simulink model "PMSMdetailTestbench"  (R2022b)
settings: Solver=ode1be  StartTime=0.0  StopTime=400  FixedStep=electricDrive.PmsmControlParams.Ts  RelTol=1e-3  EnableMultiTasking=on
PreLoadFcn:
  | PMSMSystemParamsPopl;
  | load WaterProperties.mat;
  | PMSMthermalParams;
StopFcn:
  | ee_addSimlogTimeStamp(bdroot)
undefined symbols (not defined in the file): electricDrive, p
libraries: fl_lib x71, nesl_utility x25, fl_ps_legacy_lib x23, ee_lib x4, eeTransforms x2, batteryecm_lib x1, autolibshared x1, eePmsmCurrentController x1, eePmsmFwController x1, simulink x1, eePmsmCurrentReferenceGen x1, eeVelocityController x1
(part 2 of 2)

== system PMSMdetailTestbench/Cooling System/Sensing Temperature ==
  Pressure & Temperature Sensor (TL) : fl_lib/Thermal Liquid/Sensors/Pressure & Temperature Sensor (TL)
      settings: InternalSimscapePortConfiguration="{\"Bottom\":[],\"Left\":[{\"id\":\"A\",\"label\":\"A\",\"type\":\"foundation.thermal_liquid.thermal_liquid\"}],\"Right\":[{\"id\":\"B\",\"label\":\"B\",\"type\":\"foundation.thermal_liquid.thermal_liquid\"},{\"id\":\"P\",\"label\":\"P\",\"type\":\"output\"},{\"id\":\"T\",\"label\":\"T\",\"type\":\"output\"}],\"Top\":[]}"
  TLRef : fl_lib/Thermal Liquid/Elements/Absolute Reference (TL)
  T : PMIOPort  Side=Right
  A : PMIOPort  Port=2  Side=Left
  connections:
  Pressure & Temperature Sensor (TL)/RConn3 -- T/RConn1
  TLRef/LConn1 -- Pressure & Temperature Sensor (TL)/RConn1
  A/RConn1 -- Pressure & Temperature Sensor (TL)/LConn1

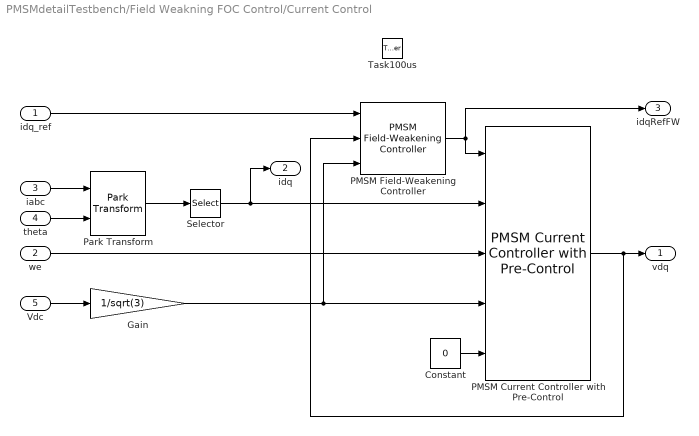
== system PMSMdetailTestbench/Field Weakning FOC Control/Current Control ==
  idq_ref : Inport
  we : Inport  Port=2
  iabc : Inport  Port=3
  theta : Inport  Port=4
  Vdc : Inport  Port=5
  Task100us : TriggerPort  TriggerType=function-call  VariantControl=Variant  PortDimensions=1
  Constant : Constant  Value=0  SampleTime=-1
  Gain : Gain  Gain=1/sqrt(3)
  PMSM Current Controller with Pre-Control : eePmsmCurrentController/PMSM Current Controller with Pre-Control  Kp_id=electricDrive.PmsmControlParams.Kp_id  Ki_id=electricDrive.PmsmControlParams.Ki_id  Kaw_id=1  Kp_iq=electricDrive.PmsmControlParams.Kp_iq  Ki_iq=electricDrive.PmsmControlParams.Ki_iq  Kaw_iq=1  Ts=-1  Tsd=electricDrive.PmsmControlParams.Tsi  AxisPrio=Q-axis  ActZC=on  ActFF=on  idVect=[-200, 0, 200]  iqVect=[-200, 0, 200]  LdMatrix=electricDrive.Ld * ones(3, 3)  LqMatrix=electricDrive.Lq * ones(3, 3)  psimMatrix=electricDrive.PmsmControlParams.psim * ones(3, 3)
  PMSM Field-Weakening Controller : eePmsmFwController/PMSM Field-Weakening Controller  Mth=0.95  Kfw=electricDrive.PmsmControlParams.Ki_fw  Kaw=electricDrive.PmsmControlParams.Kaw_fw  Ts=-1
  Park Transform : eeTransforms/Park Transform  AxisAlignment=Q-axis  PowerInvariant=off
  Selector : Selector  InputPortWidth=3  IndexOptions=Index vector (dialog)  Indices=[1 2]  OutputSizes=1
  vdq : Outport  VectorParamsAs1DForOutWhenUnconnected=off
  idq : Outport  Port=2  VectorParamsAs1DForOutWhenUnconnected=off
  idqRefFW : Outport  Port=3  VectorParamsAs1DForOutWhenUnconnected=off
  wires:
  Vdc/1 -> Gain/1
  iabc/1 -> Park Transform/1
  we/1 -> PMSM Current Controller with Pre-Control/3
  theta/1 -> Park Transform/2
  Constant/1 -> PMSM Current Controller with Pre-Control/5
  Selector/1 -> PMSM Current Controller with Pre-Control/2, idq/1
  Gain/1 -> PMSM Field-Weakening Controller/3, PMSM Current Controller with Pre-Control/4
  Park Transform/1 -> Selector/1
  PMSM Field-Weakening Controller/1 -> idqRefFW/1, PMSM Current Controller with Pre-Control/1
  PMSM Current Controller with Pre-Control/1 -> PMSM Field-Weakening Controller/2, vdq/1
  idq_ref/1 -> PMSM Field-Weakening Controller/1

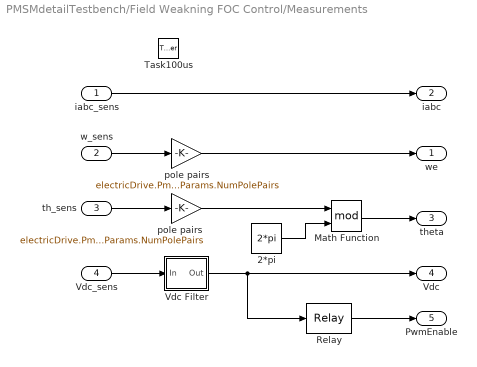
== system PMSMdetailTestbench/Field Weakning FOC Control/Measurements ==
  iabc_sens : Inport
  w_sens : Inport  Port=2
  th_sens : Inport  Port=3
  Vdc_sens : Inport  Port=4
  Task100us : TriggerPort  TriggerType=function-call  VariantControl=Variant  PortDimensions=1
  2*pi : Constant  Value=2*pi  SampleTime=-1
  Math Function : Math  Operator=mod  SignedPower=on
  Relay : Relay  OnSwitchValue=200  OffSwitchValue=100
  Vdc Filter : Subsystem  mask(Discrete first-order filter (Low-pass)){T=0.005, Ts=1e-4}
      mask prompts: T "Time constant (s):"; Ts "Sample time (s):"
      mask help: This block implements a discrete low-pass filter. To calculate the coefficients, the block discretises a continuous low-pass filter using the Tustin method.
      mask init:
      | num = [ Ts/(2*T + Ts), Ts/(2*T + Ts)];
      | den = [ 1, -(2*T - Ts)/(2*T + Ts)];
  pole pairs : Gain  Gain=electricDrive.PmsmParams.NumPolePairs
  "pole pairs " : Gain  Gain=electricDrive.PmsmParams.NumPolePairs
  we : Outport  VectorParamsAs1DForOutWhenUnconnected=off
  iabc : Outport  Port=2  VectorParamsAs1DForOutWhenUnconnected=off
  theta : Outport  Port=3  VectorParamsAs1DForOutWhenUnconnected=off
  Vdc : Outport  Port=4  VectorParamsAs1DForOutWhenUnconnected=off
  PwmEnable : Outport  Port=5  VectorParamsAs1DForOutWhenUnconnected=off
  wires:
  pole pairs/1 -> we/1
  Vdc_sens/1 -> Vdc Filter/1(In)
  th_sens/1 -> "pole pairs "/1
  w_sens/1 -> pole pairs/1
  iabc_sens/1 -> iabc/1
  "pole pairs "/1 -> Math Function/1
  2*pi/1 -> Math Function/2
  Math Function/1 -> theta/1
  Relay/1 -> PwmEnable/1
  Vdc Filter/1(Out) -> Relay/1, Vdc/1

== system PMSMdetailTestbench/Field Weakning FOC Control/Outer Loop Control ==
  RPMReq : Inport
  we : Inport  Port=2
  Vdc : Inport  Port=3
  Task1ms : TriggerPort  TriggerType=function-call  VariantControl=Variant  PortDimensions=1
  Constant : Constant  Value=0  SampleTime=-1
  PMSM Current Reference Generator : eePmsmCurrentReferenceGen/PMSM Current Reference Generator  Vnom=electricDrive.Vnom  Pmax=electricDrive.Pmax  Tmax=electricDrive.Tmax  Ts=-1  RefType=Zero d-axis control  rpmVec=[0, 3000]  TqVec=[-100, 0, 100]  VdcVec=[300, 350]  PWMMode=SVM: space vector modulation  ModFactor=1  idMatrix=zeros(2,3,2)  iqMatrix=zeros(2,3,2)  p=electricDrive.PmsmParams.NumPolePairs  psim=electricDrive.PmsmControlParams.psim  Ld=0.00024  Lq=0.00029  Rs=0.01  RefExpEnable=0
  Velocity Controller : eeVelocityController/Velocity Controller  CtrlType=P-PI control  Kp_w=electricDrive.PmsmControlParams.Kp_omega  Ki_w=electricDrive.PmsmControlParams.Ki_omega  Kv_w=electricDrive.PmsmControlParams.Kp_omega  Kaw_w=100  Ts=-1  Tsd=electricDrive.PmsmControlParams.Tso  ActZC=on
  elec->mech : Gain  Gain=1/electricDrive.PmsmParams.NumPolePairs
  rpm->rad/s : Gain  Gain=(pi/30)
  idqRef : Outport  VectorParamsAs1DForOutWhenUnconnected=off
  Tq_ref : Outport  Port=2  VectorParamsAs1DForOutWhenUnconnected=off
  Tq_lim : Outport  Port=3  VectorParamsAs1DForOutWhenUnconnected=off
  wires:
  rpm->rad/s/1 -> Velocity Controller/1
  Velocity Controller/1 -> PMSM Current Reference Generator/1
  RPMReq/1 -> rpm->rad/s/1
  we/1 -> elec->mech/1
  Vdc/1 -> PMSM Current Reference Generator/3
  PMSM Current Reference Generator/2 -> Tq_ref/1, Velocity Controller/3
  PMSM Current Reference Generator/3 -> Tq_lim/1
  elec->mech/1 -> PMSM Current Reference Generator/2, Velocity Controller/2
  Constant/1 -> Velocity Controller/4
  PMSM Current Reference Generator/1 -> idqRef/1

== system PMSMdetailTestbench/Scopes/Modulation index ==
  vdq : Inport
  Vdc : Inport  Port=2
  Gain1 : Gain  Gain=1/sqrt(3)
  Math Function : Math  Operator=square  SignedPower=on
  Prevent division by 0 : Subsystem
  Product : Product  Inputs=*/
  Rate Transition4 : RateTransition  OutPortSampleTime=electricDrive.PmsmControlParams.Tsi
  Rate Transition5 : RateTransition  OutPortSampleTime=electricDrive.PmsmControlParams.Tsi
  Sqrt : Sqrt
  Sum of Elements : Sum  Inputs=+
  M : Outport  VectorParamsAs1DForOutWhenUnconnected=off
  wires:
  Sum of Elements/1 -> Sqrt/1
  Vdc/1 -> Rate Transition4/1
  Sqrt/1 -> Product/1
  Math Function/1 -> Sum of Elements/1
  Product/1 -> M/1
  Prevent division by 0/1(OUT) -> Product/2
  vdq/1 -> Rate Transition5/1
  Rate Transition4/1 -> Gain1/1
  Gain1/1 -> Prevent division by 0/1(IN)
  Rate Transition5/1 -> Math Function/1

== system PMSMdetailTestbench/Test Environment/Bus ==
  In : Inport
  Wi : Inport  Port=2
  Br : Inport  Port=3
  Bus Creator : BusCreator  Inputs=3
  b : Outport  VectorParamsAs1DForOutWhenUnconnected=off
  wires:
  Wi/1 -> Bus Creator/2  "Wind speed"
  Bus Creator/1 -> b/1
  Br/1 -> Bus Creator/3  "Brake pedal"
  In/1 -> Bus Creator/1  "Incline"

== system PMSMdetailTestbench/Vehicle Dynamics/Brake Torque ==
  Pedal : Inport
  Force for max pedal deflection : Gain  Gain=100
  Ideal Torque Sensor : fl_lib/Mechanical/Mechanical Sensors/Ideal Torque Sensor
  Ideal Torque Source : fl_lib/Mechanical/Mechanical Sources/Ideal Torque Source
  MRRef : fl_lib/Mechanical/Rotational Elements/Mechanical Rotational Reference
  PS-Simulink Converter : nesl_utility/PS-Simulink Converter  PhysicalDomain=network_engine_domain  SubClassName=ps_output  LeftPortType=input  RightPortType=output  PseudoPeriodic=off  Frequencies=[]  VectorFormat=inherit  Unit=inherit  AffineConversion=off
  Paddle travel : TransferFcn  Numerator=[4]  Denominator=[2 1]
  Scope : Scope
  Simulink-PS Converter1 : nesl_utility/Simulink-PS Converter  PhysicalDomain=network_engine_domain  SubClassName=ps_input  LeftPortType=input  RightPortType=output  PseudoPeriodic=off  Frequencies=[]  NoiseDistribution=none  NoiseParameters=[]  Unit=N*m  AffineConversion=off  FilteringAndDerivatives=zero  SimscapeFilterOrder=1  InputFilterTimeConstant=0.001  UdotUserProvided=1
  Torque per unit brake pedal force : Gain  Gain=7.5
  R : PMIOPort  Side=Right
  wires:
  Pedal/1 -> Paddle travel/1
  Force for max pedal deflection/1 -> Torque per unit brake pedal force/1
  PS-Simulink Converter/1 -> Scope/1
  Torque per unit brake pedal force/1 -> Simulink-PS Converter1/1
  Paddle travel/1 -> Force for max pedal deflection/1
  connections:
  MRRef/LConn1 -- Ideal Torque Source/RConn2
  Ideal Torque Source/LConn1 -- Ideal Torque Sensor/RConn1
  Ideal Torque Source/RConn1 -- Simulink-PS Converter1/RConn1
  Ideal Torque Sensor/LConn1 -- R/RConn1
  PS-Simulink Converter/LConn1 -- Ideal Torque Sensor/RConn2

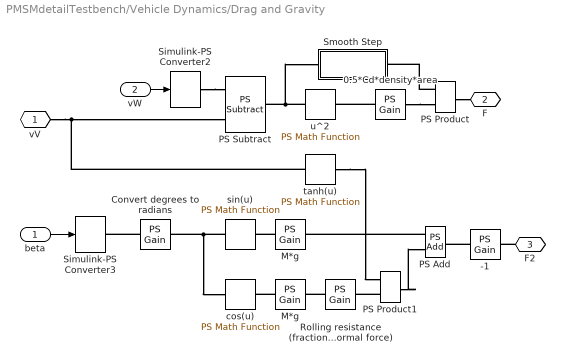
== system PMSMdetailTestbench/Vehicle Dynamics/Drag and Gravity ==
  beta : Inport
  vW : Inport  Port=2
  " M*g " : fl_ps_legacy_lib/Legacy Physical Signals/Functions/PS Gain  gain=electricDrive.VehicleParams.vehicle_mass*electricDrive.gravity
  -1 : fl_ps_legacy_lib/Legacy Physical Signals/Functions/PS Gain  gain=-1
  0.5*Cd*density*area : fl_ps_legacy_lib/Legacy Physical Signals/Functions/PS Gain  gain=0.5*electricDrive.drag_coefficient*electricDrive.air_density*electricDrive.VehicleParams.Frontalarea
  "Convert degrees to radians " : fl_ps_legacy_lib/Legacy Physical Signals/Functions/PS Gain  gain=pi/180
  M*g : fl_ps_legacy_lib/Legacy Physical Signals/Functions/PS Gain  gain=electricDrive.VehicleParams.vehicle_mass*electricDrive.gravity
  PS Add : fl_ps_legacy_lib/Legacy Physical Signals/Functions/PS Add
      settings: InternalSimscapePortConfiguration="{\"Bottom\":[],\"Left\":[{\"id\":\"I1\",\"label\":\"\",\"type\":\"input\"},{\"id\":\"I2\",\"label\":\"\",\"type\":\"input\"}],\"Right\":[{\"id\":\"O\",\"label\":\"\",\"type\":\"output\"}],\"Top\":[]}"
  PS Product : fl_ps_legacy_lib/Legacy Physical Signals/Functions/PS Product
  PS Product1 : fl_ps_legacy_lib/Legacy Physical Signals/Functions/PS Product
  PS Subtract : fl_ps_legacy_lib/Legacy Physical Signals/Functions/PS Subtract
  "Rolling resistance (fraction of normal force) " : fl_ps_legacy_lib/Legacy Physical Signals/Functions/PS Gain  gain=electricDrive.VehicleParams.rolling_res_ratio
  Simulink-PS Converter2 : nesl_utility/Simulink-PS Converter  PhysicalDomain=network_engine_domain  SubClassName=ps_input  LeftPortType=input  RightPortType=output  PseudoPeriodic=off  Frequencies=[]  NoiseDistribution=none  NoiseParameters=[]  Unit=N*m  AffineConversion=off  FilteringAndDerivatives=zero  SimscapeFilterOrder=1  InputFilterTimeConstant=0.001  UdotUserProvided=1
  Simulink-PS Converter3 : nesl_utility/Simulink-PS Converter  PhysicalDomain=network_engine_domain  SubClassName=ps_input  LeftPortType=input  RightPortType=output  PseudoPeriodic=off  Frequencies=[]  NoiseDistribution=none  NoiseParameters=[]  Unit=N*m  AffineConversion=off  FilteringAndDerivatives=zero  SimscapeFilterOrder=1  InputFilterTimeConstant=0.001  UdotUserProvided=1
  Smooth Step : Subsystem
  cos(u) : fl_ps_legacy_lib/Legacy Physical Signals/Functions/PS Math Function  fcn_choice=2
      settings: InternalSimscapePortConfiguration="{\"Bottom\":[],\"Left\":[{\"id\":\"I\",\"label\":\"\",\"type\":\"input\"}],\"Right\":[{\"id\":\"O\",\"label\":\"\",\"type\":\"output\"}],\"Top\":[]}"
  sin(u) : fl_ps_legacy_lib/Legacy Physical Signals/Functions/PS Math Function  fcn_choice=1
      settings: InternalSimscapePortConfiguration="{\"Bottom\":[],\"Left\":[{\"id\":\"I\",\"label\":\"\",\"type\":\"input\"}],\"Right\":[{\"id\":\"O\",\"label\":\"\",\"type\":\"output\"}],\"Top\":[]}"
  tanh(u) : fl_ps_legacy_lib/Legacy Physical Signals/Functions/PS Math Function  fcn_choice=10
      settings: InternalSimscapePortConfiguration="{\"Bottom\":[],\"Left\":[{\"id\":\"I\",\"label\":\"\",\"type\":\"input\"}],\"Right\":[{\"id\":\"O\",\"label\":\"\",\"type\":\"output\"}],\"Top\":[]}"
  u^2 : fl_ps_legacy_lib/Legacy Physical Signals/Functions/PS Math Function  fcn_choice=7
      settings: InternalSimscapePortConfiguration="{\"Bottom\":[],\"Left\":[{\"id\":\"I\",\"label\":\"\",\"type\":\"input\"}],\"Right\":[{\"id\":\"O\",\"label\":\"\",\"type\":\"output\"}],\"Top\":[]}"
  vV : PMIOPort  Side=Left
  F : PMIOPort  Port=2  Side=Left
  F2 : PMIOPort  Port=3  Side=Left
  wires:
  vW/1 -> Simulink-PS Converter2/1
  beta/1 -> Simulink-PS Converter3/1
  connections:
  vV/RConn1 -- tanh(u)/LConn1 -- PS Subtract/LConn1
  Simulink-PS Converter2/RConn1 -- PS Subtract/LConn2
  u^2/LConn1 -- Smooth Step/LConn1 -- PS Subtract/RConn1
  0.5*Cd*density*area/LConn1 -- u^2/RConn1
  0.5*Cd*density*area/RConn1 -- PS Product/LConn2
  PS Product/RConn1 -- F/RConn1
  PS Product/LConn1 -- Smooth Step/RConn1
  "Convert degrees to radians "/LConn1 -- Simulink-PS Converter3/RConn1
  sin(u)/LConn1 -- "Convert degrees to radians "/RConn1 -- cos(u)/LConn1
  M*g/LConn1 -- sin(u)/RConn1
  " M*g "/LConn1 -- cos(u)/RConn1
  "Rolling resistance (fraction of normal force) "/LConn1 -- " M*g "/RConn1
  PS Product1/LConn2 -- "Rolling resistance (fraction of normal force) "/RConn1
  PS Add/LConn1 -- M*g/RConn1
  PS Product1/RConn1 -- PS Add/LConn2
  -1/LConn1 -- PS Add/RConn1
  F2/RConn1 -- -1/RConn1
  tanh(u)/RConn1 -- PS Product1/LConn1

== system PMSMdetailTestbench/Vehicle Dynamics/Sensing Speed ==
  MTRef : fl_lib/Mechanical/Translational Elements/Mechanical Translational Reference
  Motion Sensor : fl_lib/Mechanical/Mechanical Sensors/Ideal Translational Motion Sensor  reference=foundation.enum.MeasurementReference.difference  acceleration_port=false  velocity_port=true  position_port=true  offset=0 m
  PS-Simulink Converter3 : nesl_utility/PS-Simulink Converter  PhysicalDomain=network_engine_domain  SubClassName=ps_output  LeftPortType=input  RightPortType=output  PseudoPeriodic=off  Frequencies=[]  VectorFormat=1-D array  Unit=mph  AffineConversion=off
  R : PMIOPort  Side=Left
  w : PMIOPort  Port=2  Side=Right
  tag scope: vSpd=global
  wires:
  PS-Simulink Converter3/1 -> [vSpd]  "Vehicle Speed"
  connections:
  R/RConn1 -- Motion Sensor/LConn1
  MTRef/LConn1 -- Motion Sensor/RConn1
  Motion Sensor/RConn2 -- PS-Simulink Converter3/LConn1 -- w/RConn1

== system PMSMdetailTestbench/ Motor Thermal/Air_HTC_calculation/Rotor side  HTC ==
  Abs : Abs  SaturateOnIntegerOverflow=off
  Gain4 : Gain  Gain=0.75
  PS-Simulink Converter5 : nesl_utility/PS-Simulink Converter  PhysicalDomain=network_engine_domain  SubClassName=ps_output  LeftPortType=input  RightPortType=output  PseudoPeriodic=off  Frequencies=[]  VectorFormat=inherit  Unit=inherit  AffineConversion=off
  Sqrt : Sqrt
  Unit Delay3 : UnitDelay  SampleTime=-1  HasFrameUpgradeWarning=on
  RPM : PMIOPort  Side=Left
  Output : Outport
  wires:
  Gain4/1 -> Output/1
  Sqrt/1 -> Gain4/1
  Unit Delay3/1 -> Abs/1
  Abs/1 -> Sqrt/1
  PS-Simulink Converter5/1 -> Unit Delay3/1
  connections:
  RPM/RConn1 -- PS-Simulink Converter5/LConn1

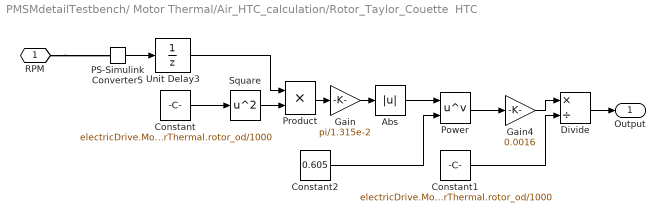
== system PMSMdetailTestbench/ Motor Thermal/Air_HTC_calculation/Rotor_Taylor_Couette  HTC ==
  Abs : Abs  SaturateOnIntegerOverflow=off
  Constant : Constant  Value=electricDrive.MotorThermal.rotor_od/1000
  Constant1 : Constant  Value=electricDrive.MotorThermal.rotor_od/1000
  Constant2 : Constant  Value=0.605
  Divide : Product  Inputs=*/
  Gain : Gain  Gain=pi/1.315e-2
  Gain4 : Gain  Gain=0.0016
  PS-Simulink Converter5 : nesl_utility/PS-Simulink Converter  PhysicalDomain=network_engine_domain  SubClassName=ps_output  LeftPortType=input  RightPortType=output  PseudoPeriodic=off  Frequencies=[]  VectorFormat=inherit  Unit=inherit  AffineConversion=off
  Power : Math  Operator=pow
  Product : Product
  Square : Math  Operator=square
  Unit Delay3 : UnitDelay  SampleTime=-1  HasFrameUpgradeWarning=on
  RPM : PMIOPort  Side=Left
  Output : Outport
  wires:
  Power/1 -> Gain4/1
  Unit Delay3/1 -> Product/1
  PS-Simulink Converter5/1 -> Unit Delay3/1
  Product/1 -> Gain/1
  Square/1 -> Product/2
  Constant/1 -> Square/1
  Gain4/1 -> Divide/1
  Constant1/1 -> Divide/2
  Divide/1 -> Output/1
  Gain/1 -> Abs/1
  Abs/1 -> Power/1
  Constant2/1 -> Power/2
  connections:
  RPM/RConn1 -- PS-Simulink Converter5/LConn1

== system PMSMdetailTestbench/ Motor Thermal/Loss Re-distribution/Iron Loss ==
  Hmot_s : Inport
  Gain1 : Gain  Gain=electricDrive.MotorThermal.vFractBridge
  Gain2 : Gain  Gain=electricDrive.MotorThermal.vFractTooth
  Unit Delay : UnitDelay  SampleTime=-1  HasFrameUpgradeWarning=on
  st : Outport
  rt : Outport  Port=2
  wires:
  Hmot_s/1 -> Gain1/1, Unit Delay/1  "Iron_Loss"
  Gain1/1 -> rt/1
  Unit Delay/1 -> Gain2/1
  Gain2/1 -> st/1

== system PMSMdetailTestbench/ Motor Thermal/Loss Re-distribution/Subsystem ==
  Heat Flow Rate Sensor : fl_lib/Thermal/Thermal Sensors/Heat Flow Rate Sensor
  PS-Simulink Converter1 : nesl_utility/PS-Simulink Converter  PhysicalDomain=network_engine_domain  SubClassName=ps_output  LeftPortType=input  RightPortType=output  PseudoPeriodic=off  Frequencies=[]  VectorFormat=inherit  Unit=inherit  AffineConversion=off
  Temperature Source : fl_lib/Thermal/Thermal Sources/Temperature Source  temperature=298.15 K
  Hmot : PMIOPort  Side=Left
  Hmot_Cu : Outport
  wires:
  PS-Simulink Converter1/1 -> Hmot_Cu/1
  connections:
  Heat Flow Rate Sensor/RConn1 -- PS-Simulink Converter1/LConn1
  Hmot/RConn1 -- Heat Flow Rate Sensor/LConn1
  Temperature Source/LConn1 -- Heat Flow Rate Sensor/RConn2

== system PMSMdetailTestbench/ Motor Thermal/Loss Re-distribution/Subsystem1 ==
  Heat Flow Rate Sensor : fl_lib/Thermal/Thermal Sensors/Heat Flow Rate Sensor
  PS-Simulink Converter1 : nesl_utility/PS-Simulink Converter  PhysicalDomain=network_engine_domain  SubClassName=ps_output  LeftPortType=input  RightPortType=output  PseudoPeriodic=off  Frequencies=[]  VectorFormat=inherit  Unit=inherit  AffineConversion=off
  Temperature Source : fl_lib/Thermal/Thermal Sources/Temperature Source  temperature=298.15 K
  Hmot : PMIOPort  Side=Left
  Hmot_Fe : Outport
  wires:
  PS-Simulink Converter1/1 -> Hmot_Fe/1
  connections:
  Heat Flow Rate Sensor/RConn1 -- PS-Simulink Converter1/LConn1
  Hmot/RConn1 -- Heat Flow Rate Sensor/LConn1
  Temperature Source/LConn1 -- Heat Flow Rate Sensor/RConn2

== system PMSMdetailTestbench/ Motor Thermal/Loss Re-distribution/Subsystem2 ==
  Heat Flow Rate Sensor : fl_lib/Thermal/Thermal Sensors/Heat Flow Rate Sensor
  PS-Simulink Converter1 : nesl_utility/PS-Simulink Converter  PhysicalDomain=network_engine_domain  SubClassName=ps_output  LeftPortType=input  RightPortType=output  PseudoPeriodic=off  Frequencies=[]  VectorFormat=inherit  Unit=inherit  AffineConversion=off
  Temperature Source : fl_lib/Thermal/Thermal Sources/Temperature Source  temperature=298.15 K
  Hmot : PMIOPort  Side=Left
  Hmot_Cu : Outport
  wires:
  PS-Simulink Converter1/1 -> Hmot_Cu/1
  connections:
  Heat Flow Rate Sensor/RConn1 -- PS-Simulink Converter1/LConn1
  Hmot/RConn1 -- Heat Flow Rate Sensor/LConn1
  Temperature Source/LConn1 -- Heat Flow Rate Sensor/RConn2

== system PMSMdetailTestbench/ Motor Thermal/Loss Re-distribution/Subsystem3 ==
  Heat Flow Rate Sensor : fl_lib/Thermal/Thermal Sensors/Heat Flow Rate Sensor
  PS-Simulink Converter1 : nesl_utility/PS-Simulink Converter  PhysicalDomain=network_engine_domain  SubClassName=ps_output  LeftPortType=input  RightPortType=output  PseudoPeriodic=off  Frequencies=[]  VectorFormat=inherit  Unit=inherit  AffineConversion=off
  Temperature Source : fl_lib/Thermal/Thermal Sources/Temperature Source  temperature=298.15 K
  Hmot : PMIOPort  Side=Left
  Hmot_Cu : Outport
  wires:
  PS-Simulink Converter1/1 -> Hmot_Cu/1
  connections:
  Heat Flow Rate Sensor/RConn1 -- PS-Simulink Converter1/LConn1
  Hmot/RConn1 -- Heat Flow Rate Sensor/LConn1
  Temperature Source/LConn1 -- Heat Flow Rate Sensor/RConn2

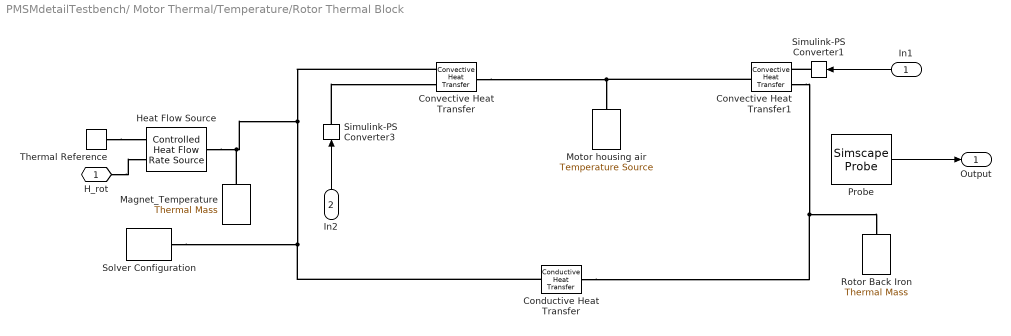
== system PMSMdetailTestbench/ Motor Thermal/Temperature/Rotor Thermal Block ==
  In1 : Inport
  In2 : Inport  Port=2
  Conductive Heat Transfer : fl_lib/Thermal/Thermal Elements/Conductive Heat Transfer  thermal_type=foundation.enum.ConstantVariableTabulated.Constant  wall_geometry=foundation.enum.ConductionWallGeometry.Cylindrical  area=1e-4 m^2  thickness=0.1 m  d_in=0.005 m  d_out=electricDrive.MotorThermal.rotor_od m  L=electricDrive.MotorThermal.rotorStackLength m  th_cond_min=10 W/(K*m)  th_cond=electricDrive.IronThConductivity W/(K*m)  th_cond_TLU=[413, 401, 392, 383, 371, 357, 342] W/(K*m)  temp_TLU=[200, 273, 400, 600, 800, 1000, 1200] K  T_specify=off  T_priority=None  T=0 K  T_nominal_specify=off  T_nominal_unit=K  T_nominal_value=1  Q_specify=off  Q_priority=None  Q=0 W  Q_nominal_specify=off  Q_nominal_unit=W  Q_nominal_value=1
  Convective Heat Transfer : fl_lib/Thermal/Thermal Elements/Convective Heat Transfer  thermal_type=foundation.enum.constant_variable.variable  area=electricDrive.MotorThermal.RotorAreaCyl m^2  heat_tr_coeff=10 W/(K*m^2)  min_heat_tr_coeff=1e-3 W/(K*m^2)  T_specify=off  T_priority=None  T=0 K  T_nominal_specify=off  T_nominal_unit=K  T_nominal_value=1  Q_specify=off  Q_priority=None  Q=0 W  Q_nominal_specify=off  Q_nominal_unit=W  Q_nominal_value=1
      settings: InternalSimscapePortConfiguration="{\"Bottom\":[],\"Left\":[{\"id\":\"A\",\"label\":\"A\",\"type\":\"foundation.thermal.thermal\"},{\"id\":\"var_heat_tr_coeff\",\"label\":\"K\",\"type\":\"input\"}],\"Right\":[{\"id\":\"B\",\"label\":\"B\",\"type\":\"foundation.thermal.thermal\"}],\"Top\":[]}"
  Convective Heat Transfer1 : fl_lib/Thermal/Thermal Elements/Convective Heat Transfer  thermal_type=foundation.enum.constant_variable.variable  area=electricDrive.MotorThermal.RotorAreaER m^2  heat_tr_coeff=20 W/(K*m^2)  min_heat_tr_coeff=1e-3 W/(K*m^2)  T_specify=off  T_priority=None  T=0 K  T_nominal_specify=off  T_nominal_unit=K  T_nominal_value=1  Q_specify=off  Q_priority=None  Q=0 W  Q_nominal_specify=off  Q_nominal_unit=W  Q_nominal_value=1
      settings: InternalSimscapePortConfiguration="{\"Bottom\":[],\"Left\":[{\"id\":\"A\",\"label\":\"A\",\"type\":\"foundation.thermal.thermal\"},{\"id\":\"var_heat_tr_coeff\",\"label\":\"K\",\"type\":\"input\"}],\"Right\":[{\"id\":\"B\",\"label\":\"B\",\"type\":\"foundation.thermal.thermal\"}],\"Top\":[]}"
  Heat Flow Source : fl_lib/Thermal/Thermal Sources/Controlled Heat Flow Rate Source
  "Magnet_Temperature " : fl_lib/Thermal/Thermal Elements/Thermal Mass  mass=electricDrive.MotorThermal.Bridgemass kg  sp_heat=447 J/(K*kg)  num_ports=foundation.enum.numPorts2.one  T_specify=on  T_priority=High  T=298.15 K  T_nominal_specify=off  T_nominal_unit=K  T_nominal_value=1  Q_specify=off  Q_priority=None  Q=0 W  Q_nominal_specify=off  Q_nominal_unit=W  Q_nominal_value=1
  Motor housing air : fl_lib/Thermal/Thermal Sources/Temperature Source  temperature=298.15 K
  Probe : SimscapeProbe  BoundBlock=1368  Variables={T}
  Rotor Back Iron : fl_lib/Thermal/Thermal Elements/Thermal Mass  mass=electricDrive.MotorThermal.RotorBackIronMass kg  sp_heat=447 J/(K*kg)  num_ports=foundation.enum.numPorts2.one  T_specify=on  T_priority=High  T=298.15 K  T_nominal_specify=off  T_nominal_unit=K  T_nominal_value=1  Q_specify=off  Q_priority=None  Q=0 W  Q_nominal_specify=off  Q_nominal_unit=W  Q_nominal_value=1
  Simulink-PS Converter1 : nesl_utility/Simulink-PS Converter  PhysicalDomain=network_engine_domain  SubClassName=ps_input  LeftPortType=input  RightPortType=output  PseudoPeriodic=off  Frequencies=[]  NoiseDistribution=none  NoiseParameters=[]  Unit=W/(K* m^2)  AffineConversion=off  FilteringAndDerivatives=provide  SimscapeFilterOrder=1  InputFilterTimeConstant=0.001  UdotUserProvided=0
  Simulink-PS Converter3 : nesl_utility/Simulink-PS Converter  PhysicalDomain=network_engine_domain  SubClassName=ps_input  LeftPortType=input  RightPortType=output  PseudoPeriodic=off  Frequencies=[]  NoiseDistribution=none  NoiseParameters=[]  Unit=W/(K* m^2)  AffineConversion=off  FilteringAndDerivatives=provide  SimscapeFilterOrder=1  InputFilterTimeConstant=0.001  UdotUserProvided=0
  Solver Configuration : nesl_utility/Solver Configuration  PhysicalDomain=network_engine_domain  SubClassName=solver  LeftPortType=input  RightPortType=generic  Tones=[]  Harmonics=[]  SimulateNoise=off  Profile=off  UseLocalSampling=off  EnableSwitchedLinearOptims=on  FrequencyDomain=off  UseCCode=off  RelTol=0.001  AbsTol=0.001  MinStep=1e-09  ToWorkspace=off  RevertToSquareIcSolve=off  NumHomotopyIterations=100  PhasorMode=off  PhasorModeNumHarmonics=1  ConsistencySolver=NEWTON_XTOL_AFTER_FTOL  IndexReductionMethod=DerivativeReplacement  DoDC=off  ResidualTolerance=1e-09  ConsistencyTolSource=GLOBAL  ConsistencyAbsTol=0.001  ConsistencyRelTol=0.001  ConsistencyTolFactor=0.001  UseLocalSolver=on  LocalSolverChoice=NE_BACKWARD_EULER_ADVANCER  ResolveIndetEquations=on  FunctionEvalNumThread=1  LocalSolverSampleTime=electricDrive.dt  DoFixedCost=on  MaxNonlinIter=3  MaxModeIter=2  ComputeImpulses=off  ImpulseIterations=2  LinearAlgebra=auto  LinearAlgebraNumThread=0  EquationFormulation=NE_TIME_EF  DelaysMemoryBudget=1024  AutomaticFiltering=on  FilteringTimeConstant=0.001  PartitionStorageMethod=AS_NEEDED  PartitionMemoryBudget=1024  PartitionMethod=ROBUST
  Thermal Reference : fl_lib/Thermal/Thermal Elements/Thermal Reference
  H_rot : PMIOPort  Side=Right
  Output : Outport
  wires:
  In2/1 -> Simulink-PS Converter3/1
  Probe/1 -> Output/1
  In1/1 -> Simulink-PS Converter1/1
  connections:
  Thermal Reference/LConn1 -- Heat Flow Source/RConn2
  Conductive Heat Transfer/RConn1 -- Convective Heat Transfer1/LConn1 -- Rotor Back Iron/LConn1
  Convective Heat Transfer1/RConn1 -- Convective Heat Transfer/RConn1 -- Motor housing air/LConn1
  Heat Flow Source/LConn1 -- Convective Heat Transfer/LConn1 -- Conductive Heat Transfer/LConn1 -- Solver Configuration/RConn1 -- "Magnet_Temperature "/LConn1
  Simulink-PS Converter3/RConn1 -- Convective Heat Transfer/LConn2
  H_rot/RConn1 -- Heat Flow Source/RConn1
  Simulink-PS Converter1/RConn1 -- Convective Heat Transfer1/LConn2

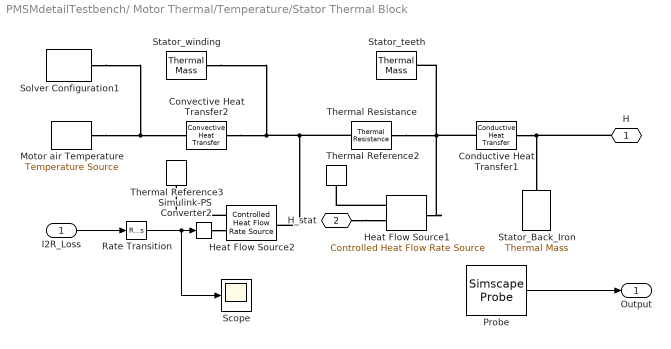
== system PMSMdetailTestbench/ Motor Thermal/Temperature/Stator Thermal Block ==
  I2R_Loss : Inport
  Conductive Heat Transfer1 : fl_lib/Thermal/Thermal Elements/Conductive Heat Transfer  thermal_type=foundation.enum.ConstantVariableTabulated.Constant  wall_geometry=foundation.enum.ConductionWallGeometry.Cylindrical  area=1e-4 m^2  thickness=0.1 m  d_in=electricDrive.MotorThermal.StatorRootDia m  d_out=electricDrive.MotorThermal.stator_od m  L=electricDrive.MotorThermal.rotorStackLength m  th_cond_min=10 W/(K*m)  th_cond=50 W/(K*m)  th_cond_TLU=[413, 401, 392, 383, 371, 357, 342] W/(K*m)  temp_TLU=[200, 273, 400, 600, 800, 1000, 1200] K  T_specify=off  T_priority=None  T=0 K  T_nominal_specify=off  T_nominal_unit=K  T_nominal_value=1  Q_specify=off  Q_priority=None  Q=0 W  Q_nominal_specify=off  Q_nominal_unit=W  Q_nominal_value=1
  Convective Heat Transfer2 : fl_lib/Thermal/Thermal Elements/Convective Heat Transfer  thermal_type=foundation.enum.constant_variable.constant  area=electricDrive.MotorThermal.StatorWindingOhArea m^2  heat_tr_coeff=1 W/(K*m^2)  min_heat_tr_coeff=1e-3 W/(K*m^2)  T_specify=off  T_priority=None  T=0 K  T_nominal_specify=off  T_nominal_unit=K  T_nominal_value=1  Q_specify=off  Q_priority=None  Q=0 W  Q_nominal_specify=off  Q_nominal_unit=W  Q_nominal_value=1
  Heat Flow Source1 : fl_lib/Thermal/Thermal Sources/Controlled Heat Flow Rate Source
  Heat Flow Source2 : fl_lib/Thermal/Thermal Sources/Controlled Heat Flow Rate Source
  Motor air Temperature : fl_lib/Thermal/Thermal Sources/Temperature Source  temperature=90 degC
  Probe : SimscapeProbe  BoundBlock=1401  Variables={T}
  Rate Transition : RateTransition
  Scope : Scope
  Simulink-PS Converter2 : nesl_utility/Simulink-PS Converter  PhysicalDomain=network_engine_domain  SubClassName=ps_input  LeftPortType=input  RightPortType=output  PseudoPeriodic=off  Frequencies=[]  NoiseDistribution=none  NoiseParameters=[]  Unit=W  AffineConversion=off  FilteringAndDerivatives=provide  SimscapeFilterOrder=1  InputFilterTimeConstant=0.001  UdotUserProvided=0
  Solver Configuration1 : nesl_utility/Solver Configuration  PhysicalDomain=network_engine_domain  SubClassName=solver  LeftPortType=input  RightPortType=generic  Tones=[]  Harmonics=[]  SimulateNoise=off  Profile=off  UseLocalSampling=off  EnableSwitchedLinearOptims=on  FrequencyDomain=off  UseCCode=off  RelTol=0.001  AbsTol=0.001  MinStep=1e-09  ToWorkspace=off  RevertToSquareIcSolve=off  NumHomotopyIterations=100  PhasorMode=off  PhasorModeNumHarmonics=1  ConsistencySolver=NEWTON_XTOL_AFTER_FTOL  IndexReductionMethod=DerivativeReplacement  DoDC=off  ResidualTolerance=1e-09  ConsistencyTolSource=GLOBAL  ConsistencyAbsTol=0.001  ConsistencyRelTol=0.001  ConsistencyTolFactor=0.001  UseLocalSolver=on  LocalSolverChoice=NE_BACKWARD_EULER_ADVANCER  ResolveIndetEquations=on  FunctionEvalNumThread=1  LocalSolverSampleTime=electricDrive.dt  DoFixedCost=on  MaxNonlinIter=3  MaxModeIter=2  ComputeImpulses=off  ImpulseIterations=2  LinearAlgebra=auto  LinearAlgebraNumThread=0  EquationFormulation=NE_TIME_EF  DelaysMemoryBudget=1024  AutomaticFiltering=on  FilteringTimeConstant=0.001  PartitionStorageMethod=AS_NEEDED  PartitionMemoryBudget=1024  PartitionMethod=ROBUST
  Stator_Back_Iron : fl_lib/Thermal/Thermal Elements/Thermal Mass  mass=electricDrive.MotorThermal.StatorBackIronMass kg  sp_heat=447 J/(K*kg)  num_ports=foundation.enum.numPorts2.one  T_specify=on  T_priority=High  T=298.15 K  T_nominal_specify=off  T_nominal_unit=K  T_nominal_value=1  Q_specify=off  Q_priority=None  Q=0 W  Q_nominal_specify=off  Q_nominal_unit=W  Q_nominal_value=1
  Stator_teeth : fl_lib/Thermal/Thermal Elements/Thermal Mass  mass=electricDrive.MotorThermal.GrossToothMass kg  sp_heat=447 J/(K*kg)  num_ports=foundation.enum.numPorts2.one  T_specify=on  T_priority=High  T=298.15 K  T_nominal_specify=off  T_nominal_unit=K  T_nominal_value=1  Q_specify=off  Q_priority=None  Q=0 W  Q_nominal_specify=off  Q_nominal_unit=W  Q_nominal_value=1
  Stator_winding : fl_lib/Thermal/Thermal Elements/Thermal Mass  mass=electricDrive.MotorThermal.WindingMass kg  sp_heat=385 J/(K*kg)  num_ports=foundation.enum.numPorts2.one  T_specify=on  T_priority=High  T=298.15 K  T_nominal_specify=off  T_nominal_unit=K  T_nominal_value=1  Q_specify=off  Q_priority=None  Q=0 W  Q_nominal_specify=off  Q_nominal_unit=W  Q_nominal_value=1
  Thermal Reference2 : fl_lib/Thermal/Thermal Elements/Thermal Reference
  Thermal Reference3 : fl_lib/Thermal/Thermal Elements/Thermal Reference
  Thermal Resistance : fl_lib/Thermal/Thermal Elements/Thermal Resistance  resistance=0.005 K/W  T_specify=off  T_priority=None  T=0 K  T_nominal_specify=off  T_nominal_unit=K  T_nominal_value=1  Q_specify=off  Q_priority=None  Q=0 W  Q_nominal_specify=off  Q_nominal_unit=W  Q_nominal_value=1
  H : PMIOPort  Side=Left
  H_stat : PMIOPort  Port=2  Side=Right
  Output : Outport
  wires:
  Probe/1 -> Output/1
  I2R_Loss/1 -> Rate Transition/1
  Rate Transition/1 -> Scope/1, Simulink-PS Converter2/1
  connections:
  Conductive Heat Transfer1/RConn1 -- H/RConn1 -- Stator_Back_Iron/LConn1
  Simulink-PS Converter2/RConn1 -- Heat Flow Source2/RConn1
  Heat Flow Source1/LConn1 -- Thermal Resistance/LConn1 -- Conductive Heat Transfer1/LConn1 -- Stator_teeth/LConn1
  Stator_winding/LConn1 -- Thermal Resistance/RConn1 -- Heat Flow Source2/LConn1 -- Convective Heat Transfer2/LConn1
  Motor air Temperature/LConn1 -- Solver Configuration1/RConn1 -- Convective Heat Transfer2/RConn1
  Heat Flow Source2/RConn2 -- Thermal Reference3/LConn1
  Heat Flow Source1/RConn2 -- Thermal Reference2/LConn1
  H_stat/RConn1 -- Heat Flow Source1/RConn1

== system PMSMdetailTestbench/Cooling System/Heat Exch. Characteristic/Characteristic ==
  PS Product : fl_ps_legacy_lib/Legacy Physical Signals/Functions/PS Product
  PS Subtract : fl_ps_legacy_lib/Legacy Physical Signals/Functions/PS Subtract
  Specific dissipation (J/s/K) per unit mass flow rate : fl_ps_legacy_lib/Legacy Physical Signals/Functions/PS Gain  gain=100
  M : PMIOPort  Side=Right
  T in : PMIOPort  Port=2  Side=Right
  T Env : PMIOPort  Port=3  Side=Right
  Q : PMIOPort  Port=4  Side=Left
  connections:
  T Env/RConn1 -- PS Subtract/LConn1
  PS Product/RConn1 -- Q/RConn1
  PS Subtract/RConn1 -- PS Product/LConn1
  T in/RConn1 -- PS Subtract/LConn2
  M/RConn1 -- Specific dissipation (J/s/K) per unit mass flow rate/LConn1
  PS Product/LConn2 -- Specific dissipation (J/s/K) per unit mass flow rate/RConn1

== system PMSMdetailTestbench/Field Weakning FOC Control/Measurements/Vdc Filter ==
  In : Inport
  Discrete Transfer Fcn : DiscreteTransferFcn  Numerator=num  Denominator=den
  Out : Outport  VectorParamsAs1DForOutWhenUnconnected=off
  wires:
  Discrete Transfer Fcn/1 -> Out/1
  In/1 -> Discrete Transfer Fcn/1

== system PMSMdetailTestbench/Scopes/Modulation index/Prevent division by 0 ==
  IN : Inport
  Constant1 : Constant  Value=0.1  SampleTime=electricDrive.PmsmControlParams.Tsi
  Switch : Switch  Criteria=u2 > Threshold  Threshold=0.1  SaturateOnIntegerOverflow=off  InputSameDT=off
  OUT : Outport  VectorParamsAs1DForOutWhenUnconnected=off
  wires:
  Constant1/1 -> Switch/3
  IN/1 -> Switch/1, Switch/2
  Switch/1 -> OUT/1

== system PMSMdetailTestbench/Vehicle Dynamics/Drag and Gravity/Smooth Step ==
  1 : fl_lib/Physical Signals/Sources/PS Constant  constant=1
  2 : fl_ps_legacy_lib/Legacy Physical Signals/Functions/PS Gain  gain=2
  exp(2x) : fl_ps_legacy_lib/Legacy Physical Signals/Functions/PS Math Function  fcn_choice=3
      settings: InternalSimscapePortConfiguration="{\"Bottom\":[],\"Left\":[{\"id\":\"I\",\"label\":\"\",\"type\":\"input\"}],\"Right\":[{\"id\":\"O\",\"label\":\"\",\"type\":\"output\"}],\"Top\":[]}"
  exp(2x)+1 : fl_ps_legacy_lib/Legacy Physical Signals/Functions/PS Add
      settings: InternalSimscapePortConfiguration="{\"Bottom\":[],\"Left\":[{\"id\":\"I1\",\"label\":\"\",\"type\":\"input\"},{\"id\":\"I2\",\"label\":\"\",\"type\":\"input\"}],\"Right\":[{\"id\":\"O\",\"label\":\"\",\"type\":\"output\"}],\"Top\":[]}"
  exp(2x)-1 : fl_ps_legacy_lib/Legacy Physical Signals/Functions/PS Subtract
  tanh(x) : fl_ps_legacy_lib/Legacy Physical Signals/Functions/PS Divide
      settings: InternalSimscapePortConfiguration="{\"Bottom\":[],\"Left\":[{\"id\":\"I1\",\"label\":\"\",\"type\":\"input\"},{\"id\":\"I2\",\"label\":\"\",\"type\":\"input\"}],\"Right\":[{\"id\":\"O\",\"label\":\"\",\"type\":\"output\"}],\"Top\":[]}"
  x : PMIOPort  Side=Left
  y : PMIOPort  Port=2  Side=Right
  connections:
  y/RConn1 -- tanh(x)/RConn1
  x/RConn1 -- 2/LConn1
  exp(2x)-1/RConn1 -- tanh(x)/LConn1
  exp(2x)+1/RConn1 -- tanh(x)/LConn2
  exp(2x)+1/LConn2 -- exp(2x)-1/LConn1 -- exp(2x)/RConn1
  2/RConn1 -- exp(2x)/LConn1
  exp(2x)-1/LConn2 -- exp(2x)+1/LConn1 -- 1/RConn1

== stateflow chart PMSMdetailTestbench/Field Weakning FOC Control/Task Scheduler ==
  (default) -> (junction 23) : CLK_50us
  (junction 23) -> (junction 17)
  (junction 17) -> (junction 22) [order 2]
  (junction 17) -> (junction 22) [order 1] : [cnt%%2==0]{Task_100us_1;}
  (junction 22) -> (junction 18) [order 2]
  (junction 22) -> (junction 18) [order 1] : [cnt%%2==0]{Task_100us_2;}
  (junction 18) -> (junction 21) [order 1] : [cnt%%20==0]{Task_1ms_1;}
  (junction 18) -> (junction 21) [order 2]
  (junction 21) -> (junction 34) [order 2]
  (junction 21) -> (junction 16) [order 1] : [1]{cnt++;}
  data: cnt local int32
  events: Task_100us_1 output FUNCTION_CALL_EVENT; Task_100us_2 output FUNCTION_CALL_EVENT; Task_1ms_1 output FUNCTION_CALL_EVENT; CLK_50us input FUNCTION_CALL_EVENT
